simulink model "chapter6_MPC_DynamicModel_PlanCtrl_0424"  (Simulink 8.2)
settings: Solver=VariableStepDiscrete  StartTime=0.0  StopTime=40  FixedStep=0.01  RelTol=1e-3
libraries: Solver_SF x1, simulink x1
settings Model: Creator=xuwei  LastModifiedBy=liuho

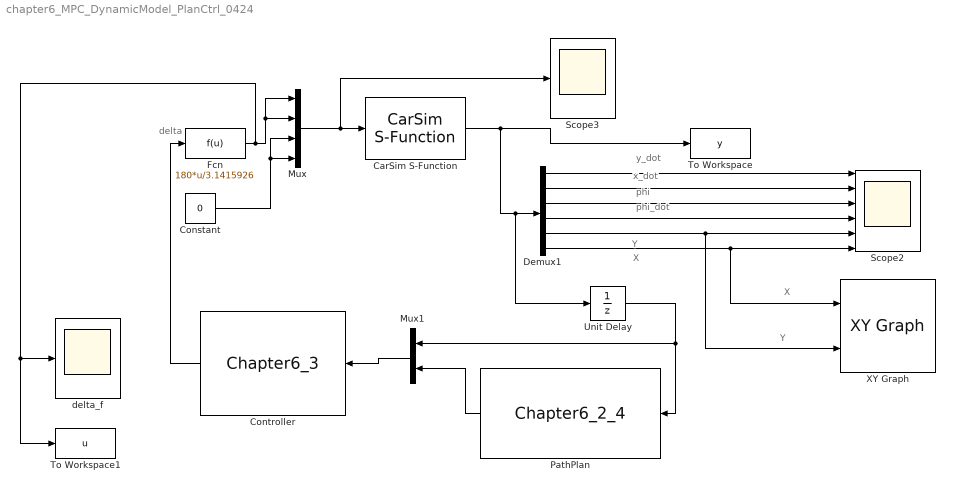
== system chapter6_MPC_DynamicModel_PlanCtrl_0424 ==
  note: delta
  note: X
  note: Y
  note: y_dot
  note: x_dot
  note: phi
  note: phi_dot
  note: Y
  note: X
  CarSim S-Function : Solver_SF/CarSim S-Function  Priority=1  VehicleCode=i_i  SIMFILE=simfile.sim
  Constant : Constant  Value=0
  Controller : S-Function  FunctionName=Chapter6_3  EnableBusSupport=off
  Demux1 : Demux  Outputs=6
  Fcn : Fcn  Expr=180*u/3.1415926
  Mux : Mux
  Mux1 : Mux  Inputs=2
  PathPlan : S-Function  FunctionName=Chapter6_2_4  EnableBusSupport=off
  Scope2 : Scope  NumInputPorts=6
      settings: TimeRange=20  YMin=-1~35~-10~-20~-4~0  YMax=1~36.5~5~20~2~200
  Scope3 : Scope
      settings: TimeRange=20  YMin=0  YMax=19  SaveName=ScopeData2
  To Workspace : ToWorkspace  VariableName=y  SampleTime=-1  SaveFormat=Structure
  To Workspace1 : ToWorkspace  VariableName=u  SampleTime=-1  SaveFormat=Structure
  Unit Delay : UnitDelay  SampleTime=-1
  XY Graph : simulink/Sinks/XY Graph  xmin=0  xmax=250  ymin=-3  ymax=6  st=-1
  delta_f : Scope
      settings: TimeRange=20  YMin=-3  YMax=3
  wires:
  CarSim S-Function/1 -> To Workspace/1, Demux1/1, Unit Delay/1
  Fcn/1 -> Mux/1, Mux/2, delta_f/1, To Workspace1/1
  Constant/1 -> Mux/4, Mux/3
  Mux/1 -> CarSim S-Function/1, Scope3/1
  Demux1/1 -> Scope2/1
  Demux1/2 -> Scope2/2
  Demux1/3 -> Scope2/3
  Demux1/4 -> Scope2/4
  Demux1/5 -> Scope2/5, XY Graph/2
  Demux1/6 -> Scope2/6, XY Graph/1
  Controller/1 -> Fcn/1
  Unit Delay/1 -> Mux1/1, PathPlan/1
  PathPlan/1 -> Mux1/2
  Mux1/1 -> Controller/1
